simulink model "TwoLevel"  (R2023b)
settings: Solver=FixedStepAuto  StartTime=0.0  StopTime=16/ffund  FixedStep=1e-6  MaxStep=1e-7  RelTol=1e-3
InitFcn:
  | fsw=5500;
  | ffund=500;
  | ma=0.5;
libraries: spsControlledVoltageSourceLib x3, spsCurrentMeasurementLib x3, spsSeriesRLCBranchLib x3, spsTriangleGeneratorLib x1, sps_lib x1
settings Model: Creator=lbocker  LastModifiedBy=enesa
settings DebuggingCC: SignalInfNanChecking=warning

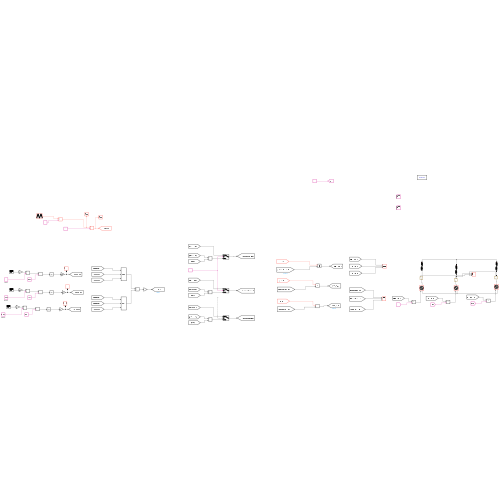
[thumbnail: Simulink's stored preview of the top-level diagram]
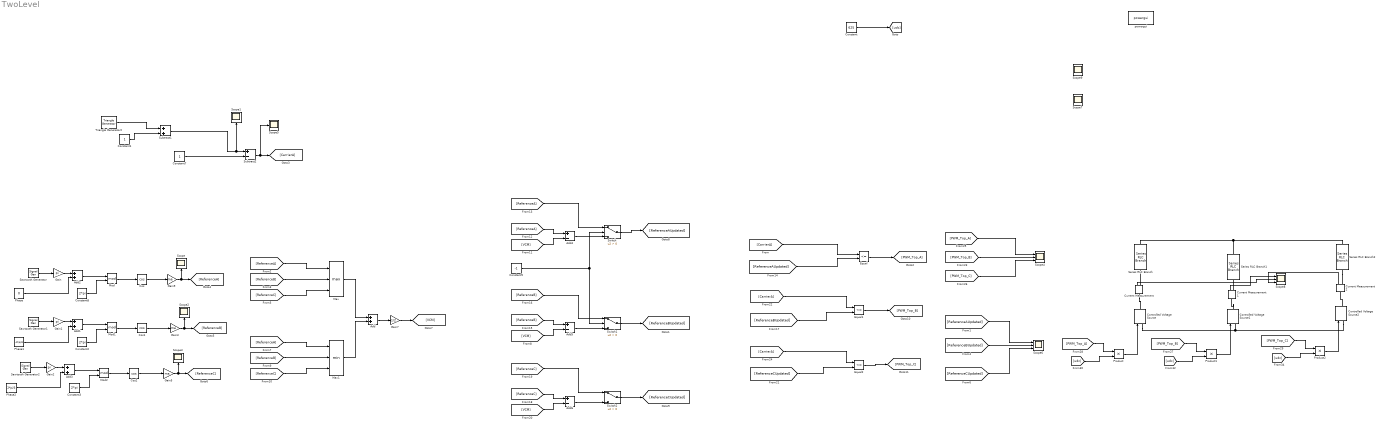
== system TwoLevel ==
  Add{,1..3} (4 alike) : Sum
  Add4 : Sum  Inputs=+-
  Add5 : Sum  Inputs=+-
  Add6 : Sum  Inputs=+-
  Constant : Constant  Value=625
  Constant1 : Constant
  Constant2 : Constant  Value=2*pi
  Constant3 : Constant  Value=2*pi
  Constant5 : Constant  Value=-1
  Constant7 : Constant
  Constant8 : Constant  Value=2*pi
  Controlled Voltage Source : spsControlledVoltageSourceLib/Controlled Voltage Source  Initialize=on  Source_Type=AC  Amplitude=0  Phase=0  Frequency=0  Measurements=None
  Controlled Voltage Source1 : spsControlledVoltageSourceLib/Controlled Voltage Source  Initialize=on  Source_Type=AC  Amplitude=0  Phase=0  Frequency=0  Measurements=None
  Controlled Voltage Source2 : spsControlledVoltageSourceLib/Controlled Voltage Source  Initialize=on  Source_Type=AC  Amplitude=0  Phase=0  Frequency=0  Measurements=None
  Cos : Trigonometry  Operator=cos
  Cos1 : Trigonometry  Operator=cos
  Cos2 : Trigonometry  Operator=cos
  Current Measurement : spsCurrentMeasurementLib/Current Measurement  PhasorSimulation=off  OutputType=Complex  PSBequivalent=0
  Current Measurement1 : spsCurrentMeasurementLib/Current Measurement  PhasorSimulation=off  OutputType=Complex  PSBequivalent=0
  Current Measurement2 : spsCurrentMeasurementLib/Current Measurement  PhasorSimulation=off  OutputType=Complex  PSBequivalent=0
  Equal : RelationalOperator  Operator=<=  OutDataTypeStr=boolean  RndMeth=Simplest  InputSameDT=off
  Equal1 : RelationalOperator  Operator=<=  OutDataTypeStr=boolean  RndMeth=Simplest  InputSameDT=off
  Equal2 : RelationalOperator  Operator=<=  OutDataTypeStr=boolean  RndMeth=Simplest  InputSameDT=off
  Gain : Gain  Gain=pi
  Gain1 : Gain  Gain=pi
  Gain2 : Gain  Gain=pi
  Gain3 : Gain  Gain=ma
  Gain5 : Gain  Gain=ma
  Gain7 : Gain  Gain=1/2
  Gain9 : Gain  Gain=ma
  Max : MinMax  Function=max  Inputs=3
  Max1 : MinMax  Inputs=3
  Mod : Math  Operator=mod
  Mod1 : Math  Operator=mod
  Mod2 : Math  Operator=mod
  Phase : Constant  Value=0
  Phase1 : Constant  Value=-2*pi/3
  Phase2 : Constant  Value=2*pi/3
  Product : Product
  Product1 : Product
  Product2 : Product
  Sawtooth Generator : SignalGenerator  WaveForm=sawtooth  Frequency=2*pi*ffund  Units=rad/sec
  Sawtooth Generator1 : SignalGenerator  WaveForm=sawtooth  Frequency=2*pi*ffund  Units=rad/sec
  Sawtooth Generator2 : SignalGenerator  WaveForm=sawtooth  Frequency=2*pi*ffund  Units=rad/sec
  Scope{,1..3,5} (5 alike) : Scope
  Scope{4,6..9} (5 alike) : Scope  NumInputPorts=3
  Series RLC Branch : spsSeriesRLCBranchLib/Series RLC Branch  LConnTagsString=__new0  RConnTagsString=__new0  BranchType=RL  Resistance=1  Inductance=1e-3  SetiL0=off  InitialCurrent=0  Capacitance=1e-6  Setx0=off  InitialVoltage=0  Measurements=None
  Series RLC Branch1 : spsSeriesRLCBranchLib/Series RLC Branch  LConnTagsString=__new0  RConnTagsString=__new0  BranchType=RL  Resistance=1  Inductance=1e-3  SetiL0=off  InitialCurrent=0  Capacitance=1e-6  Setx0=off  InitialVoltage=0  Measurements=None
  Series RLC Branch2 : spsSeriesRLCBranchLib/Series RLC Branch  LConnTagsString=__new0  RConnTagsString=__new0  BranchType=RL  Resistance=1  Inductance=1e-3  SetiL0=off  InitialCurrent=0  Capacitance=1e-6  Setx0=off  InitialVoltage=0  Measurements=None
  Subtract1 : Sum
  Subtract2 : Sum  Inputs=+-
  Switch : Switch  Criteria=u2 > Threshold  SaturateOnIntegerOverflow=off  InputSameDT=off
  Switch1 : Switch  Criteria=u2 > Threshold  SaturateOnIntegerOverflow=off  InputSameDT=off
  Switch2 : Switch  Criteria=u2 > Threshold  SaturateOnIntegerOverflow=off  InputSameDT=off
  Triangle Generator2 : spsTriangleGeneratorLib/Triangle Generator  Freq=fsw  Phase=0  Ts=1e-6
  powergui : sps_lib/powergui  Priority=1  SimulationMode=Continuous  SampleTime=50e-6  frequency=60  Iterations=50  frequencyindice=0  Pbase=100e6  ErrMax=1e-4  UnitsV=kV  UnitsW=MW  buscounter=0  FunctionMessages=off  echomessages=off  EnableUseOfTLC=off  CurrentSourceSwitches=off  DisableSnubberDevices=off  DisableRonSwitches=off  DisableVfSwitches=off  DisplayEquations=off  AutomaticDiscreteSolvers=off  SolverType=Tustin/Backward Euler (TBE)  Interpol=off  ExternalGateDelay=off  methode=off  Ts=100  x0status=blocks  SPID=on  SwTol=0  HookPort=off  NonlinearTolerance=1e-4  nMaxIteration=100  ContinueOnMaxIteration=off  RestoreLinks=warning  ResistiveCurrentMeasurement=off  Frange=[0:2:500]  Ylog=off  Xlog=on  ShowGrid=off  save=off  variable=ZData  structure=0  ZoomFFT=off  StartTime=0.0  cycles=1  DisplayStyle=1  fundamental=60  FreqAxis=off  MaxFrequency=1000  frequencyindicesteady=1  RmsSteady=1  display=off
  wires:
  Constant/1 -> [udc]
  Subtract2/1 -> Scope5/1, [CarrierA]
  Constant7/1 -> Subtract2/2
  Triangle Generator2/1 -> Subtract1/1
  Constant1/1 -> Subtract1/2
  Cos/1 -> Gain9/1
  Equal/1 -> [PWM_Top_A]
  [CarrierA] -> Equal/1
  Mod/1 -> Cos/1
  Constant8/1 -> Mod/2
  Sawtooth Generator/1 -> Gain/1
  Phase/1 -> Add2/2
  Add2/1 -> Mod/1
  Gain/1 -> Add2/1
  Add1/1 -> Mod1/1
  Sawtooth Generator1/1 -> Gain1/1
  Phase1/1 -> Add1/2
  Mod1/1 -> Cos1/1
  Gain1/1 -> Add1/1
  Constant2/1 -> Mod1/2
  Sawtooth Generator2/1 -> Gain2/1
  Gain2/1 -> Add3/1
  Constant3/1 -> Mod2/2
  Phase2/1 -> Add3/2
  Mod2/1 -> Cos2/1
  Add3/1 -> Mod2/1
  Gain9/1 -> Scope/1, [ReferenceA]
  Cos1/1 -> Gain3/1
  Gain3/1 -> Scope2/1, [ReferenceB]
  Cos2/1 -> Gain5/1
  Gain5/1 -> Scope3/1, [ReferenceC]
  [ReferenceA] -> Max/1
  [ReferenceB] -> Max/2
  [ReferenceC] -> Max/3
  [ReferenceB] -> Max1/2
  [ReferenceC] -> Max1/3
  [ReferenceA] -> Max1/1
  Max/1 -> Add/1
  Max1/1 -> Add/2
  Add/1 -> Gain7/1
  Gain7/1 -> [VCM]
  [ReferenceA] -> Add4/1
  [VCM] -> Add4/2
  Add4/1 -> Switch/3
  [ReferenceA] -> Switch/1
  Switch/1 -> [ReferenceAUpdated]
  [ReferenceAUpdated] -> Equal/2
  [ReferenceAUpdated] -> Scope6/1
  [ReferenceBUpdated] -> Scope6/2
  [ReferenceCUpdated] -> Scope6/3
  [VCM] -> Add5/2
  Add5/1 -> Switch1/3
  [ReferenceB] -> Switch1/1
  [ReferenceB] -> Add5/1
  Constant5/1 -> Switch/2, Switch1/2
  Switch1/1 -> [ReferenceBUpdated]
  [ReferenceC] -> Add6/1
  Switch2/1 -> [ReferenceCUpdated]
  [ReferenceC] -> Switch2/1
  [VCM] -> Add6/2
  Add6/1 -> Switch2/3
  ? -> Switch2/2
  [ReferenceBUpdated] -> Equal1/2
  [CarrierA] -> Equal1/1
  Equal1/1 -> [PWM_Top_B]
  [ReferenceCUpdated] -> Equal2/2
  Equal2/1 -> [PWM_Top_C]
  [CarrierA] -> Equal2/1
  [PWM_Top_A] -> Scope4/1
  [PWM_Top_B] -> Scope4/2
  [PWM_Top_C] -> Scope4/3
  Subtract1/1 -> Subtract2/1, Scope1/1
  Product/1 -> Controlled Voltage Source/1
  [PWM_Top_A] -> Product/1
  [udc] -> Product/2
  [udc] -> Product1/2
  Product1/1 -> Controlled Voltage Source1/1
  [PWM_Top_B] -> Product1/1
  [udc] -> Product2/2
  Product2/1 -> Controlled Voltage Source2/1
  [PWM_Top_C] -> Product2/1
  Current Measurement/1 -> Scope8/2
  Current Measurement1/1 -> Scope8/1
  Current Measurement2/1 -> Scope8/3
  connections:
  Controlled Voltage Source/LConn1 -- Controlled Voltage Source2/LConn1 -- Controlled Voltage Source1/LConn1
  Series RLC Branch/LConn1 -- Series RLC Branch1/LConn1 -- Series RLC Branch2/LConn1
  Current Measurement/LConn1 -- Controlled Voltage Source/RConn1
  Current Measurement/RConn1 -- Series RLC Branch/RConn1
  Controlled Voltage Source1/RConn1 -- Current Measurement1/LConn1
  Current Measurement1/RConn1 -- Series RLC Branch1/RConn1
  Controlled Voltage Source2/RConn1 -- Current Measurement2/LConn1
  Series RLC Branch2/RConn1 -- Current Measurement2/RConn1
